simulink model "Clutchless_P2_Parallel"  (R2017b)
settings: Solver=FixedStepAuto  StartTime=0.0  StopTime=length(Speed)  FixedStep=0.01  MaxStep=0.01  RelTol=1e-3  EnableMultiTasking=on
PostLoadFcn:
  | , if any(exist('dsrtsu_mdlpostloadfcn', 'file') == [2, 3, 6]), try dsrtsu_mdlpostloadfcn('Execute', bdroot); catch fprintf('Error in PostLoadFcn (dsrtsu_mdlpostloadfcn) for model "%s":\n %s\n', bdroot, lasterr); end, end,
undefined symbols (not defined in the file): Actuators, APP1_OOR, APP2_OOR, APP_Mismatch, Brk_Flt, cal, Chassis, ClutchEngag, Clutchless_HSC, eng, Engine, EngineTorqueReal, EngOverTemp, ENGTRQ_MSMCH_Degraded_CP, ENGTRQ_MSMCH_ErrCritical_CP, ENGTRQ_MSMCH_LimpHome_CP, EngTrqMismatch, ess, ESSOverTemp, g, gb, Grade, KeyPos_Flt, lib_Actuators, lib_Chassis, lib_Clutchless_HSC, lib_EMachine_2017a, lib_Sensors_2017a, LossCAN, Machine, MCUOverTemp, mot, MotDirMismatch, motor_Trq, MotOverTemp, MotTrqMismatch, mph2ms, PRNDL_Flt, RegenFault, rho, Sensors, t_amb, time, tloop, veh, Vehicle
libraries: simulink x96, EC2_libraries x6, autolibmappedmotor x3, powerlib_meascontrol x2, CalculationGallon x1, lib_DCDC x1, lib_Differential x1, lib_HVESS x1, lib_Engine x1, lib_OBC x1, Scope_new x1, lib_Transmission x1
(part 4 of 10)

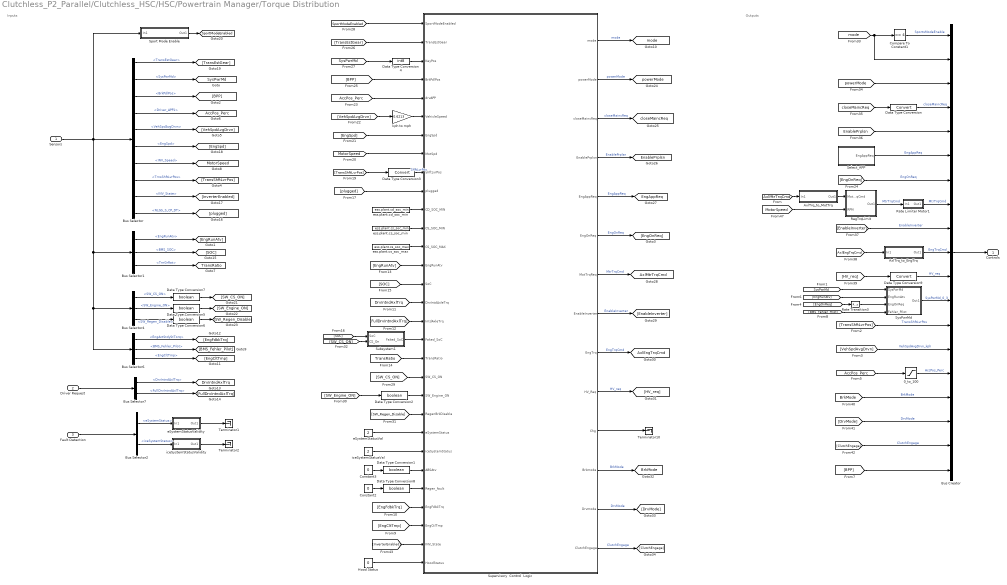
== system Clutchless_P2_Parallel/Clutchless_HSC/HSC/Powertrain Manager/Torque Distribution ==
  note: Inputs
  note: Outputs
  Sensors : Inport
  Driver Request : Inport  Port=2
  Fault Detection : Inport  Port=3
  0_to_100 : Saturate  UpperLimit=100  LowerLimit=0
  AxlTrq_to_EngTrq : Subsystem
  AxlTrq_to_MotTrq : Subsystem
  Bus Creator : BusCreator  Inputs=19
  Bus Selector : BusSelector  OutputSignals=from_CAN.fromVEH_CAN.from_TCM.TransEstGear,from_CAN.fromVEH_CAN.from_BCM.SysPwrMd,from_CAN.fromVEH_CAN.from_BCM.BrkPdlPos,from_Analog.Driver_APP1,from_CAN.fromEBCAN.from_ECM.VehSpdAvgDrvn,from_CAN.fromEBCAN.from_ECM.EngSpd,from_CAN.fromHV_CAN.from_MCU.INV_VCU_01.INV_Speed,from_CAN.fromVEH_CAN.from_TCM.TrnsShftLvrPos,from_CAN.fromHV_CAN.from_MCU.INV_VCU_01.INV_State,from_CAN.fromHV_CAN.from_OBC.NLG5_ST.NLG5_S_CP_DT
  Bus Selector1 : BusSelector  OutputSignals=from_CAN.fromEBCAN.from_ECM.EngRunAtv,from_CAN.fromHV_CAN.from_BMSHybrid.BMS_SOC,from_CAN.fromVEH_CAN.from_TCM.TrnGrRat
  Bus Selector2 : BusSelector  OutputSignals=eSystemDiagOut.eSystemStatus,iceSystemDiagOut.iceSystemStatus
  Bus Selector4 : BusSelector  OutputSignals=from_Digital.SW_CS_ON,from_Digital.SW_Engine_ON,from_Digital.SW_Regen_Disable
  Bus Selector6 : BusSelector  OutputSignals=from_CAN.fromEBCAN.from_ECM.EngActStdyStTorq,from_CAN.fromHV_CAN.from_BMSHybrid.BMS_HYB_02.BMS_Fehler_Pilot,from_CAN.fromEBCAN.from_ECM.EngCltTmp
  Bus Selector7 : BusSelector  OutputSignals=DrvIntndAxlTrq,FullDrvIntndAxlTrq
  Compare To Constant1 : simulink/Logic and Bit Operations/Compare To Constant  relop===  const=4  OutDataTypeStr=boolean
  Constant2 : Constant  Value=0
  Constant3 : Constant  Value=0
  Data Type Conversion : DataTypeConversion
  Data Type Conversion{1..2,5..8} (6 alike) : DataTypeConversion  OutDataTypeStr=boolean
  Data Type Conversion3 : DataTypeConversion
  Data Type Conversion4 : DataTypeConversion  OutDataTypeStr=int8
  Data Type Conversion9 : DataTypeConversion
  Hood Status : Constant  Value=0
  Rate Limiter Motor1 : Subsystem
  Rate Transition3 : RateTransition
  RegTrqLimit : Subsystem
  Select_APP : Subsystem
  Sport Mode Enable : Subsystem
  Subsystem1 : Subsystem
  Supervisory  Control  Logic : Stateflow chart  TreatAsAtomicUnit=on
  SysPwrMd : Subsystem
  Terminator1 : Terminator
  Terminator10 : Terminator
  Terminator2 : Terminator
  eSystemStatusVal : Constant  Value=2
  eSystemStatusValidity : Subsystem
  ess.plant.cd_soc_min : Constant  Value=ess.plant.cd_soc_min
  ess.plant.cs_soc_max : Constant  Value=ess.plant.cs_soc_max
  ess.plant.cs_soc_min : Constant  Value=ess.plant.cs_soc_min
  iceSystemStatusVal : Constant  Value=2
  iceSystemStatusValidity : Subsystem
  kph to mph : Gain  Gain=0.6213
  Controls : Outport
  tag scope: AccPos_Perc=global, AxlEngTrqCmd=global, AxlMtrTrqCmd=global, BrkMode=global, DrvIntndAxlTrq=global, EnablePrplsn=global, EngAppReq=global, MotorSpeed=global, SportModeEnabled=global, SysPwrMd=global, TransRatio=global, closeMaincReq=global, mode=global, powerMode=global
  wires:
  AxlTrq_to_MotTrq/1(Out1) -> RegTrqLimit/1(MotTrqCmd)
  [AxlMtrTrqCmd] -> AxlTrq_to_MotTrq/1(In1)
  [MotorSpeed] -> RegTrqLimit/2(RPM)
  Hood Status/1 -> Supervisory  Control  Logic/30(HoodStatus)
  [plugged] -> Supervisory  Control  Logic/10(plugged)
  AxlTrq_to_EngTrq/1(Out1) -> Bus Creator/10  "EngTrqCmd"
  [closeMaincReq] -> Data Type Conversion/1
  Compare To Constant1/1 -> Bus Creator/1  "SportsModeEnable"
  [EngRunAtv] -> SysPwrMd/2(EngRunAtv)
  [ClutchEngage] -> Bus Creator/18  "ClutchEngage"
  [BPP] -> Bus Creator/19
  [AxlEngTrqCmd] -> AxlTrq_to_EngTrq/1(In1)
  [mode] -> Compare To Constant1/1, Bus Creator/2
  [TransShftLvrPos] -> Bus Creator/13  "TransShftLvrPos"
  [DrvMode] -> Bus Creator/17  "DrvMode"
  [SysPwrMd] -> SysPwrMd/1(SysPwrMd)
  SysPwrMd/1(Out1) -> Bus Creator/12  "SysPwrMd_0_3"
  [VehSpdAvgDrvn] -> Bus Creator/14  "VehSpdAvgDrvn_kph"
  Data Type Conversion9/1 -> Bus Creator/11  "HV_req"
  [BMS_Fehler_Pilot] -> SysPwrMd/4(Fehler_Pilot)
  [EnablePrplsn] -> Bus Creator/5
  [AccPos_Perc] -> 0_to_100/1
  [EnableInverter] -> Bus Creator/9  "EnableInverter"
  [EngOnReq] -> Bus Creator/7  "EngOnReq"
  [HV_req] -> Data Type Conversion9/1
  Select_APP/1(EngAppReq) -> Bus Creator/6  "EngAppReq"
  [BrkMode] -> Bus Creator/16  "BrkMode"
  0_to_100/1 -> Bus Creator/15  "AccPos_Perc"
  [powerMode] -> Bus Creator/3
  Data Type Conversion/1 -> Bus Creator/4  "closeMaincReq"
  [EngOnReq] -> Rate Transition3/1
  Rate Transition3/1 -> SysPwrMd/3(EngOnReq)
  Bus Creator/1 -> Controls/1
  Sensors/1 -> Bus Selector/1, Bus Selector1/1, Bus Selector4/1, Bus Selector6/1, Sport Mode Enable/1(In1)
  Bus Selector/1 -> [TransEstGear]  "<TransEstGear>"
  Bus Selector/2 -> [SysPwrMd]  "<SysPwrMd>"
  Bus Selector/3 -> [BPP]  "<BrkPdlPos>"
  Bus Selector/4 -> [AccPos_Perc]  "<Driver_APP1>"
  Bus Selector/5 -> [VehSpdAvgDrvn]  "<VehSpdAvgDrvn>"
  Bus Selector/6 -> [EngSpd]  "<EngSpd>"
  Bus Selector/7 -> [MotorSpeed]  "<INV_Speed>"
  Bus Selector/9 -> [InverterEnabled]  "<INV_State>"
  Bus Selector1/1 -> [EngRunAtv]  "<EngRunAtv>"
  Bus Selector/8 -> [TransShftLvrPos]  "<TrnsShftLvrPos>"
  Bus Selector1/3 -> [TransRatio]  "<TrnGrRat>"
  Fault Detection/1 -> Bus Selector2/1
  Bus Selector2/1 -> eSystemStatusValidity/1(In1)  "<eSystemStatus>"
  Bus Selector2/2 -> iceSystemStatusValidity/1(In1)  "<iceSystemStatus>"
  Bus Selector4/3 -> Data Type Conversion6/1  "<SW_Regen_Disable>"
  Bus Selector4/1 -> Data Type Conversion7/1  "<SW_CS_ON>"
  Bus Selector4/2 -> Data Type Conversion5/1  "<SW_Engine_ON>"
  eSystemStatusValidity/1(Out1) -> Terminator1/1
  iceSystemStatusValidity/1(Out1) -> Terminator2/1
  Bus Selector/10 -> [plugged]  "<NLG5_S_CP_DT>"
  Data Type Conversion5/1 -> [SW_Engine_ON]
  Data Type Conversion6/1 -> [SW_Regen_Disable]
  Bus Selector6/1 -> [EngFdbkTrq]  "<EngActStdyStTorq>"
  Bus Selector6/2 -> [BMS_Fehler_Pilot]  "<BMS_Fehler_Pilot>"
  Bus Selector6/3 -> [EngCltTmp]  "<EngCltTmp>"
  Bus Selector7/2 -> [FullDrvIntndAxlTrq]  "<FullDrvIntndAxlTrq>"
  Sport Mode Enable/1(Out1) -> [SportModeEnabled]
  Bus Selector1/2 -> [SOC]  "<BMS_SOC>"
  Data Type Conversion7/1 -> [SW_CS_ON]
  Driver Request/1 -> Bus Selector7/1
  Bus Selector7/1 -> [DrvIntndAxlTrq]  "<DrvIntndAxlTrq>"
  Supervisory  Control  Logic/14(ClutchEngage) -> [ClutchEngage]  "ClutchEngage"
  Supervisory  Control  Logic/13(Drvmode) -> [DrvMode]  "DrvMode"
  Supervisory  Control  Logic/10(HV_Req) -> [HV_req]  "HV_req"
  Supervisory  Control  Logic/9(EngTrq) -> [AxlEngTrqCmd]  "EngTrqCmd"
  Supervisory  Control  Logic/7(MotTrqReq) -> [AxlMtrTrqCmd]  "MtrTrqCmd"
  Supervisory  Control  Logic/6(EngOnReq) -> [EngOnReq]  "EngOnReq"
  [SW_CS_ON] -> Subsystem1/2(CS_On)
  [SW_Regen_Disable] -> Supervisory  Control  Logic/22(RegenBrkDisable)
  [SW_CS_ON] -> Supervisory  Control  Logic/20(SW_CS_ON)
  [SportModeEnabled] -> Supervisory  Control  Logic/1(SportModeEnabled)
  Data Type Conversion4/1 -> Supervisory  Control  Logic/3(KeyPos)
  [SysPwrMd] -> Data Type Conversion4/1
  [TransEstGear] -> Supervisory  Control  Logic/2(TransEstGear)
  [BPP] -> Supervisory  Control  Logic/4(BrkPdlPos)
  [AccPos_Perc] -> Supervisory  Control  Logic/5(drvAPP)
  [VehSpdAvgDrvn] -> kph to mph/1
  [EngSpd] -> Supervisory  Control  Logic/7(EngSpd)
  [TransShftLvrPos] -> Data Type Conversion3/1
  [SOC] -> Subsystem1/1(SoC)
  [SOC] -> Supervisory  Control  Logic/15(SoC)
  [TransRatio] -> Supervisory  Control  Logic/19(TransRatio)
  [EngRunAtv] -> Supervisory  Control  Logic/14(EngRunAtv)
  [EngFdbkTrq] -> Supervisory  Control  Logic/27(EngFdbkTrq)
  [EngCltTmp] -> Supervisory  Control  Logic/28(EngCtlTmp)
  [MotorSpeed] -> Supervisory  Control  Logic/8(MotSpd)
  Supervisory  Control  Logic/5(EngAppReq) -> [EngAppReq]  "EngAppReq"
  eSystemStatusVal/1 -> Supervisory  Control  Logic/23(eSystemStatus)
  iceSystemStatusVal/1 -> Supervisory  Control  Logic/24(iceSystemStatus)
  Data Type Conversion8/1 -> Supervisory  Control  Logic/26(Regen_fault)
  Supervisory  Control  Logic/12(Brkmode) -> [BrkMode]  "BrkMode"
  Subsystem1/1(Faked_SoC) -> Supervisory  Control  Logic/18(Faked_SoC)
  Data Type Conversion1/1 -> Supervisory  Control  Logic/25(ABSAtv)
  Constant3/1 -> Data Type Conversion1/1
  [FullDrvIntndAxlTrq] -> Supervisory  Control  Logic/17(IntdAxleTrq)
  [DrvIntndAxlTrq] -> Supervisory  Control  Logic/16(DrvIntdAxleTrq)
  Supervisory  Control  Logic/11(Chg) -> Terminator10/1
  Constant2/1 -> Data Type Conversion8/1
  kph to mph/1 -> Supervisory  Control  Logic/6(VehicleSpeed)
  Data Type Conversion3/1 -> Supervisory  Control  Logic/9(ShftLvrPos)  "ShftLvrPos"
  Supervisory  Control  Logic/1(mode) -> [mode]  "mode"
  Supervisory  Control  Logic/2(powerMode) -> [powerMode]  "powerMode"
  Supervisory  Control  Logic/3(closeMaincReq) -> [closeMaincReq]  "closeMaincReq"
  Supervisory  Control  Logic/4(EnablePrplsn) -> [EnablePrplsn]  "EnablePrplsn"
  Supervisory  Control  Logic/8(EnableInverter) -> [EnableInverter]  "EnableInverter"
  ess.plant.cs_soc_max/1 -> Supervisory  Control  Logic/13(CS_SOC_MAX)
  ess.plant.cs_soc_min/1 -> Supervisory  Control  Logic/12(CS_SOC_MIN)
  ess.plant.cd_soc_min/1 -> Supervisory  Control  Logic/11(CD_SOC_MIN)
  [SW_Engine_ON] -> Data Type Conversion2/1
  Data Type Conversion2/1 -> Supervisory  Control  Logic/21(SW_Engine_ON)
  [InverterEnabled] -> Supervisory  Control  Logic/29(INV_State)
  RegTrqLimit/1(Out1) -> Rate Limiter Motor1/1(In1)  "MtrTrqCmd"
  Rate Limiter Motor1/1(Out1) -> Bus Creator/8  "MtrTrqCmd"

== system Clutchless_P2_Parallel/Sensors/CAN/EBCAN/BMS_Antrieb ==
  In1 : Inport
  Bus Creator : BusCreator  Inputs=2
  Bus Selector : BusSelector  OutputSignals=NMH_BMS,ISO_Hybrid_01_Resp
  ISO_Hybrid_01_Resp : Subsystem
  NMH_BMS : Subsystem
  Out1 : Outport
  wires:
  Bus Selector/2 -> ISO_Hybrid_01_Resp/1(In1)  "<ISO_Hybrid_01_Resp>"
  Bus Creator/1 -> Out1/1
  ISO_Hybrid_01_Resp/1(Out1) -> Bus Creator/2
  NMH_BMS/1(Out1) -> Bus Creator/1
  Bus Selector/1 -> NMH_BMS/1(In1)  "<NMH_BMS>"
  In1/1 -> Bus Selector/1

== system Clutchless_P2_Parallel/Sensors/CAN/EBCAN/CCM ==
  In1 : Inport
  Bus Creator : BusCreator  Inputs=2
  Bus Selector : BusSelector  OutputSignals=NMH_BMS,ISO_Hybrid_01_Resp
  ISO_Hybrid_01_Resp : Subsystem
  NMH_BMS : Subsystem
  Out1 : Outport
  wires:
  In1/1 -> Bus Selector/1
  Bus Selector/1 -> NMH_BMS/1(In1)  "<NMH_BMS>"
  NMH_BMS/1(Out1) -> Bus Creator/1
  ISO_Hybrid_01_Resp/1(Out1) -> Bus Creator/2
  Bus Creator/1 -> Out1/1
  Bus Selector/2 -> ISO_Hybrid_01_Resp/1(In1)  "<ISO_Hybrid_01_Resp>"

== system Clutchless_P2_Parallel/Sensors/CAN/EBCAN/ECM ==
  In1 : Inport
  Bus Creator : BusCreator  Inputs=7
  Bus Selector : BusSelector  OutputSignals=Sensors_to_ECM.EngActStdyStTorq_Nm,Sensors_to_ECM.EngSpd_RPM,ECM_to_Actuators.VehSpdAvgDrvn,ECM_to_Actuators.EngRunAtv,ECM_to_Actuators.Eng_Temp,ECM_to_Actuators.ECM_RollingAliveCnt
  Data Type Conversion{1..6} (6 alike) : DataTypeConversion
  ETEI_Engine_Torque_Status : Subsystem
  Ground : Ground
  PPEI_Engine_General_Status_4 : Subsystem
  PPEI_Engine_General_Status_6 : Subsystem
  PPEI_Vehicle_Speed_and_Distance : Subsystem
  PTEI_Engine_Torque_Status : Subsystem
  Out1 : Outport
  wires:
  Data Type Conversion1/1 -> Bus Creator/4  "EngRunAtv"
  Data Type Conversion3/1 -> Bus Creator/2  "EngSpd"
  PPEI_Engine_General_Status_6/1(Out1) -> Bus Creator/7
  Data Type Conversion6/1 -> PPEI_Engine_General_Status_6/1(In1)
  PPEI_Engine_General_Status_4/1(Out1) -> Bus Creator/6
  Data Type Conversion5/1 -> PPEI_Engine_General_Status_4/1(In1)
  PTEI_Engine_Torque_Status/1(Out1) -> Bus Creator/5
  Ground/1 -> PTEI_Engine_Torque_Status/1(In1)
  Bus Selector/4 -> Data Type Conversion1/1  "<EngRunAtv>"
  Bus Creator/1 -> Out1/1
  PPEI_Vehicle_Speed_and_Distance/1(Out1) -> Bus Creator/3
  ETEI_Engine_Torque_Status/1(Out1) -> Bus Creator/1
  Data Type Conversion4/1 -> PPEI_Vehicle_Speed_and_Distance/1(In1)
  Bus Selector/2 -> Data Type Conversion3/1  "<EngSpd_RPM>"
  Data Type Conversion2/1 -> ETEI_Engine_Torque_Status/1(In1)
  In1/1 -> Bus Selector/1
  Bus Selector/1 -> Data Type Conversion2/1  "<EngActStdyStTorq_Nm>"
  Bus Selector/3 -> Data Type Conversion4/1  "<VehSpdAvgDrvn>"
  Bus Selector/5 -> Data Type Conversion5/1  "<Eng_Temp>"
  Bus Selector/6 -> Data Type Conversion6/1  "<ECM_RollingAliveCnt>"

== system Clutchless_P2_Parallel/Sensors/CAN/HV_CAN/BMS_Hybrid ==
  In1 : Inport
  BMS_HYB_02 : Subsystem
  BMS_HYB_03 : Subsystem
  BMS_HYB_04 : Subsystem
  Bus Creator : BusCreator  Inputs=6
  Bus Selector : BusSelector  OutputSignals=BMS_HYB_02,BMS_HYB_04,BMS_HYB_03,BMS_HYB_02.BMS_Fehler_Isolation,BMS_HYB_06.BMS_Temperatur,BMS_HYB_02.BMS_Fehler_HS_verschweisst
  Data Type Conversion : DataTypeConversion
  Data Type Conversion1 : DataTypeConversion
  Data Type Conversion2 : DataTypeConversion
  Out1 : Outport
  wires:
  Data Type Conversion2/1 -> Bus Creator/6  "BMS_Fehler_HS_verschweisst"
  Bus Selector/5 -> Data Type Conversion/1  "<BMS_Temperatur>"
  Bus Selector/4 -> Data Type Conversion1/1  "<BMS_Fehler_Isolation>"
  BMS_HYB_03/1(Out1) -> Bus Creator/3
  Bus Selector/3 -> BMS_HYB_03/1(In1)  "<BMS_HYB_03>"
  BMS_HYB_04/1(Out1) -> Bus Creator/2
  BMS_HYB_02/1(Out1) -> Bus Creator/1
  Bus Creator/1 -> Out1/1
  Bus Selector/2 -> BMS_HYB_04/1(In1)  "<BMS_HYB_04>"
  Bus Selector/1 -> BMS_HYB_02/1(In1)  "<BMS_HYB_02>"
  In1/1 -> Bus Selector/1
  Data Type Conversion/1 -> Bus Creator/5  "BMS_Temperatur"
  Data Type Conversion1/1 -> Bus Creator/4  "BMS_Fehler_Isolation"
  Bus Selector/6 -> Data Type Conversion2/1  "<BMS_Fehler_HS_verschweisst>"

== system Clutchless_P2_Parallel/Sensors/CAN/HV_CAN/MCU ==
  In1 : Inport
  Bus Creator : BusCreator  Inputs=6
  Bus Creator1 : BusCreator  Inputs=2
  Bus Creator2 : BusCreator  Inputs=2
  Bus Selector : BusSelector  OutputSignals=Sensors_to_MCU.mot_spd_out,Sensors_to_MCU.mot_crr_out,MCU_to _Actuator.InverterEnabled,MCU_to _Actuator.MotTrqFdbck,MCU_to _Actuator.D3_Power_On_Timer,Sensors_to_MCU.mot_volt_in
  Bus Selector1 : BusSelector  OutputSignals=Sensors_to_MCU.mcu_temp,Sensors_to_MCU.mot_temp
  Data Type Conversion{1..5,7..9} (8 alike) : DataTypeConversion
  In2 : InportShadow
  Out1 : Outport
  wires:
  In1/1 -> Bus Selector/1
  Bus Selector/6 -> Data Type Conversion9/1  "<mot_volt_in>"
  Bus Selector/4 -> Data Type Conversion7/1  "<MotTrqFdbck>"
  Bus Selector/5 -> Data Type Conversion8/1  "<D3_Power_On_Timer>"
  Bus Creator/1 -> Bus Creator1/1  "INV_VCU_01"
  Data Type Conversion3/1 -> Bus Creator/3  "INV_State"
  Data Type Conversion2/1 -> Bus Creator/2  "INV_CurrentHV"
  Data Type Conversion1/1 -> Bus Creator/1  "INV_Speed"
  Bus Selector/3 -> Data Type Conversion3/1  "<InverterEnabled>"
  Bus Selector/2 -> Data Type Conversion2/1  "<mot_crr_out>"
  Bus Selector/1 -> Data Type Conversion1/1  "<mot_spd_out>"
  Data Type Conversion7/1 -> Bus Creator/4  "INV_OutputTorque"
  Data Type Conversion8/1 -> Bus Creator/5  "MessageCounter_200"
  Data Type Conversion9/1 -> Bus Creator/6  "INV_VoltageHV"
  Data Type Conversion4/1 -> Bus Creator2/1  "INV_InverterTemperature"
  Bus Selector1/2 -> Data Type Conversion5/1  "<mot_temp>"
  Data Type Conversion5/1 -> Bus Creator2/2  "INV_ElectricMachineTemperature"
  Bus Selector1/1 -> Data Type Conversion4/1  "<mcu_temp>"
  In2/1 -> Bus Selector1/1
  Bus Creator2/1 -> Bus Creator1/2  "INV_VCU_04"
  Bus Creator1/1 -> Out1/1

== system Clutchless_P2_Parallel/Sensors/CAN/HV_CAN/OBC ==
  In1 : Inport
  Bus Creator : BusCreator  Inputs=5
  Bus Selector : BusSelector  OutputSignals=NLG5_ACT_I,NLG5_ACT_II,NLG5_ERR,NLG5_ST,NLG5_TEMP
  NLG5_ACT_I : Subsystem
  NLG5_ACT_II : Subsystem
  NLG5_ERR : Subsystem
  NLG5_ST : Subsystem
  NLG5_TEMP : Subsystem
  Out1 : Outport
  wires:
  In1/1 -> Bus Selector/1
  Bus Selector/1 -> NLG5_ACT_I/1(In1)  "<NLG5_ACT_I>"
  NLG5_ACT_I/1(Out1) -> Bus Creator/1
  Bus Selector/2 -> NLG5_ACT_II/1(In1)  "<NLG5_ACT_II>"
  NLG5_ACT_II/1(Out1) -> Bus Creator/2
  NLG5_ERR/1(Out1) -> Bus Creator/3
  Bus Selector/3 -> NLG5_ERR/1(In1)  "<NLG5_ERR>"
  Bus Selector/4 -> NLG5_ST/1(In1)  "<NLG5_ST>"
  NLG5_ST/1(Out1) -> Bus Creator/4
  Bus Selector/5 -> NLG5_TEMP/1(In1)  "<NLG5_TEMP>"
  NLG5_TEMP/1(Out1) -> Bus Creator/5
  Bus Creator/1 -> Out1/1

== system Clutchless_P2_Parallel/Sensors/CAN/VEH_CAN/BCM ==
  In1 : Inport
  Bus Creator : BusCreator  Inputs=2
  Bus Selector : BusSelector  OutputSignals=SysPwrMd,BrkPdlPos
  Data Type Conversion : DataTypeConversion
  Data Type Conversion1 : DataTypeConversion
  PPEI_Brake_Apply_Status : Subsystem
  PPEI_Platfrom_General_Status : Subsystem
  Out1 : Outport
  wires:
  Data Type Conversion1/1 -> PPEI_Brake_Apply_Status/1(In1)
  Data Type Conversion/1 -> PPEI_Platfrom_General_Status/1(In1)
  Bus Creator/1 -> Out1/1
  PPEI_Brake_Apply_Status/1(Out1) -> Bus Creator/2
  PPEI_Platfrom_General_Status/1(Out1) -> Bus Creator/1
  Bus Selector/2 -> Data Type Conversion1/1  "<BrkPdlPos>"
  Bus Selector/1 -> Data Type Conversion/1  "<SysPwrMd>"
  In1/1 -> Bus Selector/1

== system Clutchless_P2_Parallel/Sensors/CAN/VEH_CAN/EBCM ==
  In1 : Inport
  Bus Selector : BusSelector  OutputSignals=PPEI_Chassis_General_Status_1.BrkPdlDrvAppPrsDetcd
  Constant : Constant  OutDataTypeStr=boolean
  PPEI_Chassis_General_Status_1 : Subsystem
  Terminator : Terminator
  Out1 : Outport
  wires:
  Constant/1 -> PPEI_Chassis_General_Status_1/1(In1)
  In1/1 -> Bus Selector/1
  PPEI_Chassis_General_Status_1/1(Out1) -> Out1/1
  Bus Selector/1 -> Terminator/1  "<BrkPdlDrvAppPrsDetcd>"

== system Clutchless_P2_Parallel/Sensors/CAN/VEH_CAN/ICCM ==
  In1 : Inport
  Out1 : Outport
  wires:
  In1/1 -> Out1/1

== system Clutchless_P2_Parallel/Sensors/CAN/VEH_CAN/TCM ==
  In1 : Inport
  Bus Creator : BusCreator  Inputs=4
  Bus Selector : BusSelector  OutputSignals=TCM_to _Actuator.TransEstGear,TCM_to _Actuator.LockupCmd,TCM_to _Actuator.TrnsShftLvrPos,Sensors_to_TCM.gb_trq_ratio
  Data Type Conversion{,1..3} (4 alike) : DataTypeConversion
  Out1 : Outport
  wires:
  Data Type Conversion/1 -> Bus Creator/1  "TransEstGear"
  Bus Creator/1 -> Out1/1
  In1/1 -> Bus Selector/1
  Data Type Conversion1/1 -> Bus Creator/2  "TrnsTrqCnvCltCmndMd"
  Data Type Conversion2/1 -> Bus Creator/3  "TrnsShftLvrPos"
  Data Type Conversion3/1 -> Bus Creator/4  "TrnGrRat"
  Bus Selector/1 -> Data Type Conversion/1  "<TransEstGear>"
  Bus Selector/2 -> Data Type Conversion1/1  "<LockupCmd>"
  Bus Selector/3 -> Data Type Conversion2/1  "<TrnsShftLvrPos>"
  Bus Selector/4 -> Data Type Conversion3/1  "<gb_trq_ratio>"

== system Clutchless_P2_Parallel/Camaro Plant Model/E-Machine/IMG Plant/Electric Machine/Calculate Mot Efficiency, MotPwrMech, and, MotPwrElec1 ==
  note: Pelec_req = Pmech_req*Eff^k,
      | k = -1 if Trq >= 0,
      | k = 1 if Trq < 0
  MotSpd : Inport
  MotTrqAct : Inport  Port=2
  -1 : Gain  Gain=8
  "-1 when + 1 when - " : Gain  Gain=-1
  -2 : Gain  Gain=tloop
  2-D Lookup Table : Lookup_n-D  BreakpointsForDimension1=mot.plant.init.eff_trq.idx2_trq  BreakpointsForDimension2=mot.plant.init.eff_trq.idx1_spd  Table=mot.plant.init.eff_trq.map  InternalRulePriority=Speed  RndMeth=Simplest  InputSameDT=on
  Abs{,1..3} (4 alike) : Abs
  Add : Sum  Inputs=-+
  Add1 : Sum  Inputs=+-
  Constant : Constant  Value=1-0.8
  Gain2 : Gain  Gain=1/100
  MCU_WEGPmp : Constant  Value=0
  Math Function1 : Math  Operator=pow  SaturateOnIntegerOverflow=on
  Memory : Memory
  Product : Product
  Product1 : Product
  Product2 : Product
  Sign : Signum
  rad/s to rpm : Gain  Gain=30/pi
  Losses : Outport
  MCU_Heat : Outport  Port=2
  MotPwrElec : Outport  Port=3
  wires:
  -2/1 -> MCU_Heat/1
  -1/1 -> Add1/2
  Add1/1 -> -2/1
  MCU_WEGPmp/1 -> -1/1
  Abs3/1 -> Add1/1
  Product2/1 -> Abs3/1
  Constant/1 -> Product2/2
  Memory/1 -> Sign/1
  Math Function1/1 -> Product1/2
  Add/1 -> Abs2/1
  Abs2/1 -> Losses/1
  "-1 when + 1 when - "/1 -> Math Function1/2
  MotSpd/1 -> rad/s to rpm/1, Product/2
  MotTrqAct/1 -> Abs/1, Product/1, Memory/1
  Product/1 -> Product1/1, Add/1  "MotPwrMech"
  Product1/1 -> Add/2, Product2/1, MotPwrElec/1  "MotPwrElec"
  2-D Lookup Table/1 -> Gain2/1
  Gain2/1 -> Math Function1/1
  Abs/1 -> 2-D Lookup Table/1
  Sign/1 -> "-1 when + 1 when - "/1
  Abs1/1 -> 2-D Lookup Table/2
  rad/s to rpm/1 -> Abs1/1

== system Clutchless_P2_Parallel/Camaro Plant Model/E-Machine/IMG Plant/Electric Machine/MotTrqExcessTrigger1 ==
  In1 : Inport
  Bias : Bias  Bias=55
  Bias1 : Bias  Bias=25
  Constant : Constant  Value=0
  Multiport Switch : MultiPortSwitch  DataPortOrder=Zero-based contiguous
  Terminator : Terminator
  Out1 : Outport
  tag scope: MotTrqExcessTrig=global
  wires:
  Constant/1 -> Multiport Switch/1, [MotTrqExcessTrig]
  Bias1/1 -> Multiport Switch/3
  In1/1 -> Bias1/1, Bias/1, Multiport Switch/2
  Bias/1 -> Multiport Switch/4
  Multiport Switch/1 -> Out1/1
  [MotTrqExcessTrig] -> Terminator/1

== system Clutchless_P2_Parallel/Camaro Plant Model/E-Machine/IMG Plant/Electric Machine/Thermal1 ==
  Losses : Inport
  MCU_heat : Inport  Port=2
  MotInv_loop : Subsystem
  Motor Thermal : Subsystem  Commented=on
  MCU_temp_C : Outport
  motor_temp : Outport  Port=2
  wires:
  MotInv_loop/2(Out2) -> motor_temp/1
  MotInv_loop/1(Out1) -> MCU_temp_C/1
  Losses/1 -> MotInv_loop/1(In1)  "[W]"
  MCU_heat/1 -> MotInv_loop/2(In2)

== system Clutchless_P2_Parallel/Camaro Plant Model/E-Machine/IMG Plant/Electric Machine/Torque Calculation1 ==
  MotSpd : Inport
  MotTrqCmd : Inport  Port=2
  Abs : Abs
  Abs1 : Abs
  Memory : Memory
  MinMax : MinMax  Inputs=2
  Product : Product
  Sign : Signum
  "max torque " : Subsystem
  mot_trq_out : Outport
  wires:
  Product/1 -> Memory/1
  MotTrqCmd/1 -> Abs/1, Sign/1, "max torque "/1(cmd)
  Memory/1 -> mot_trq_out/1
  Abs1/1 -> MinMax/2
  Abs/1 -> MinMax/1
  MinMax/1 -> Product/2
  Sign/1 -> Product/1
  MotSpd/1 -> "max torque "/2(speed)
  "max torque "/1(max torque) -> Abs1/1

== system Clutchless_P2_Parallel/Camaro Plant Model/E-Machine/IMG Plant/Electric Machine/non-zero division1 ==
  note: and finally, the expression is: (u[1] \ u[2]) * 1 = u[1] \ u[2]
  note: (u[2]!=0) is true then returns 1
  note: if u[2] != 0, then output == u[1]\u[2]:
  note: (u[2]==0) is false then returns 0, thus (u[2]+(u[2]==0)) is equal to u[2]+0=u[2]
  note: and finally, the expression is: (u[1] \ 1) * 0 = 0
  note: (u[2]!=0) is false then returns 0
  note: if u[2] == 0, then output == 0:
  note: (u[2]==0) is true then returns 1, thus (u[2]+(u[2]==0)) is equal to 0+1=1
  note: original idea from Phil Sharer - ANL
      | original formula: u[1]\(u[2]+eps)*(u[2]!=0)
      | changes done by Gerald ZINI (dgey) - ANL (05\02\2001)
  In1 : Inport
  In2 : Inport  Port=2
  Fcn : Fcn  Expr=u[1]/(u[2]+(u[2]==0))*(u[2]!=0)
  Mux : Mux  Inputs=2
  Out1 : Outport
  wires:
  In2/1 -> Mux/2
  Fcn/1 -> Out1/1
  In1/1 -> Mux/1
  Mux/1 -> Fcn/1

== system Clutchless_P2_Parallel/Camaro Plant Model/E-Machine/IMG Plant2/Calculate Mot Efficiency, MotPwrMech, and, MotPwrElec/Lower Limit ==
  In1 : Inport
  Constant3 : Constant  Value=Lolimit
  MinMax : MinMax  Function=max  Inputs=2
  Out1 : Outport
  wires:
  MinMax/1 -> Out1/1
  Constant3/1 -> MinMax/2
  In1/1 -> MinMax/1

== system Clutchless_P2_Parallel/Camaro Plant Model/E-Machine/IMG Plant2/Calculate Mot Efficiency, MotPwrMech, and, MotPwrElec/MCUOverTemp Fault ==
  In1 : Inport
  Gain : Gain  Gain=3
  Switch : Switch  Threshold=1
  Out1 : Outport
  wires:
  Switch/1 -> Out1/1
  Gain/1 -> Switch/1
  [MCUOverTemp] -> Switch/2
  In1/1 -> Gain/1, Switch/3

== system Clutchless_P2_Parallel/Camaro Plant Model/E-Machine/IMG Plant2/Motor_Plant/Efficiency Calcs ==
  Speed_rpm : Inport
  Torq_cmd_Nm : Inport  Port=2
  Batt_volt : Inport  Port=3
  Abs1 : Abs
  Constant : Constant
  Constant1 : Constant  Value=0
  Current_consum : Product  Inputs=*/
  Efficiency Map : Lookup_n-D  BreakpointsForDimension1=mot.map.trqindex  BreakpointsForDimension2=mot.map.spdindex  Table=mot.map.eff  InternalRulePriority=Speed  RndMeth=Simplest  InputSameDT=on
  Electrical power motoring : Product  Inputs=*//
  Electrical power regen : Product  Inputs=***
  Gain : Gain  Gain=2*3.14/60
  Gain1 : Gain  Gain=-1
  MCU_eff : Constant  Value=0.97
  Mech_power : Product  Inputs=**
  MinMax : MinMax  Function=max  Inputs=2
  MinMax1 : MinMax  Function=max  Inputs=2
  Saturation : Saturate  UpperLimit=400  LowerLimit=-400
  Switch : Switch  Criteria=u2 > Threshold
  Switch1 : Switch  Criteria=u2 > Threshold  Threshold=100
  min_eff : Constant  Value=0.1
  Mot_current : Outport
  Mech_power_W : Outport  Port=2
  Elec_power_W : Outport  Port=3
  wires:
  Constant1/1 -> Switch1/3
  Switch/1 -> Switch1/1  "Elec_power_W"
  Gain1/1 -> Saturation/1  "Mot_current_A"
  Constant/1 -> MinMax1/2
  MinMax1/1 -> Current_consum/2
  Efficiency Map/1 -> MinMax/1
  Switch1/1 -> Current_consum/1, Elec_power_W/1  "Elec_power_W"
  min_eff/1 -> MinMax/2
  Electrical power motoring/1 -> Switch/1
  MCU_eff/1 -> Electrical power motoring/3, Electrical power regen/3
  Mech_power/1 -> Mech_power_W/1, Electrical power regen/1, Electrical power motoring/1  "Mech_power_W"
  Abs1/1 -> Efficiency Map/1
  Batt_volt/1 -> MinMax1/1, Switch1/2
  Gain/1 -> Mech_power/1
  Saturation/1 -> Mot_current/1  "Mot_current_A"
  Current_consum/1 -> Gain1/1
  MinMax/1 -> Electrical power regen/2, Electrical power motoring/2
  Electrical power regen/1 -> Switch/3
  Torq_cmd_Nm/1 -> Switch/2, Abs1/1, Mech_power/2
  Speed_rpm/1 -> Gain/1, Efficiency Map/2

== system Clutchless_P2_Parallel/Camaro Plant Model/E-Machine/IMG Plant2/Thermal/Motor Thermal ==
  In1 : Inport
  Add1 : Sum  Inputs=+-
  Add2 : Sum
  Divide : Product  Inputs=*/
  Lower Limit : Subsystem  mask{Lolimit=t_amb+20}
      mask prompts: Lolimit "Lower Limit"
  Memory1 : Memory
  Motor Mass : Constant  Value=mot.plant.init.motor_mass
  Product : Product  RndMeth=Zero
  "Pump " : Constant  Value=0
  Specific Heat Cap Aluminum : Constant  Value=mot.plant.init.specific_heat
  tloop : Gain  Gain=tloop
  Out1 : Outport
  wires:
  Add1/1 -> tloop/1
  In1/1 -> Add1/1
  "Pump "/1 -> Add1/2
  Motor Mass/1 -> Product/1  "kg"
  tloop/1 -> Divide/1  "J"
  Divide/1 -> Add2/1
  Lower Limit/1(Out1) -> Memory1/1, Out1/1
  Add2/1 -> Lower Limit/1(In1)
  Memory1/1 -> Add2/2
  Product/1 -> Divide/2
  Specific Heat Cap Aluminum/1 -> Product/2  "J/kg*K"

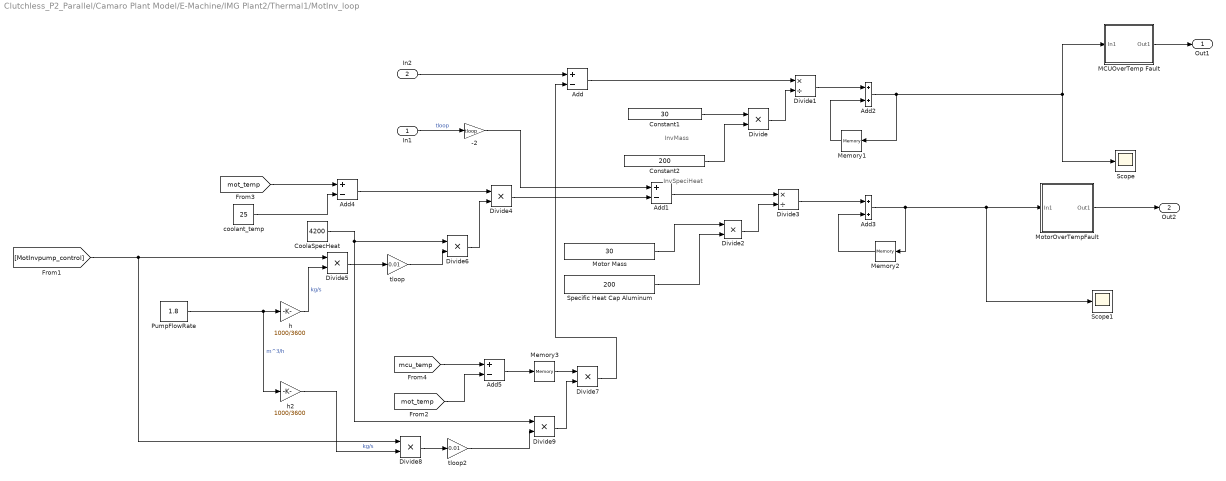
== system Clutchless_P2_Parallel/Camaro Plant Model/E-Machine/IMG Plant2/Thermal1/MotInv_loop ==
  note: InvMass
  note: InvSpeciHeat
  In1 : Inport
  In2 : Inport  Port=2
  -2 : Gain  Gain=tloop
  Add{,1,4..5} (4 alike) : Sum  Inputs=+-
  Add2 : Sum
  Add3 : Sum
  Constant1 : Constant  Value=30
  Constant2 : Constant  Value=200
  CoolaSpecHeat : Constant  Value=4200
  Divide{,2,4..9} (8 alike) : Product  Inputs=**
  Divide1 : Product  Inputs=*/
  Divide3 : Product  Inputs=*/
  MCUOverTemp Fault : Subsystem
  Memory1 : Memory  InitialCondition=25
  Memory2 : Memory  InitialCondition=25
  Memory3 : Memory
  Motor Mass : Constant  Value=30
  MotorOverTempFault : Subsystem
  PumpFlowRate : Constant  Value=1.8
  Scope : Scope
  Scope1 : Scope
  Specific Heat Cap Aluminum : Constant  Value=200
  coolant_temp : Constant  Value=25
  h : Gain  Gain=1000/3600
  h2 : Gain  Gain=1000/3600
  tloop : Gain  Gain=0.01
  tloop2 : Gain  Gain=0.01
  Out1 : Outport
  Out2 : Outport  Port=2
  wires:
  [MotInvpump_control] -> Divide5/1, Divide8/1
  -2/1 -> Add1/1
  In2/1 -> Add/1
  In1/1 -> -2/1  "tloop"
  [mot_temp] -> Add5/2
  [mcu_temp] -> Add5/1
  [mot_temp] -> Add4/1
  MotorOverTempFault/1(Out1) -> Out2/1
  MCUOverTemp Fault/1(Out1) -> Out1/1
  Memory3/1 -> Divide7/1
  Add5/1 -> Memory3/1
  Divide4/1 -> Add1/2
  tloop2/1 -> Divide9/2
  Divide8/1 -> tloop2/1
  Divide9/1 -> Divide7/2
  h2/1 -> Divide8/2  "kg/s"
  PumpFlowRate/1 -> h/1, h2/1  "m^3/h"
  CoolaSpecHeat/1 -> Divide9/1, Divide6/1
  tloop/1 -> Divide6/2
  h/1 -> Divide5/2  "kg/s"
  Divide7/1 -> Add/2
  Divide1/1 -> Add2/1
  Motor Mass/1 -> Divide2/1
  Constant2/1 -> Divide/2
  Divide2/1 -> Divide3/2
  Add2/1 -> Memory1/1, Scope/1, MCUOverTemp Fault/1(In1)
  Divide5/1 -> tloop/1
  Divide3/1 -> Add3/1
  Divide6/1 -> Divide4/2
  Add3/1 -> Memory2/1, MotorOverTempFault/1(In1), Scope1/1
  Add4/1 -> Divide4/1
  Memory2/1 -> Add3/2
  Add/1 -> Divide1/1
  Constant1/1 -> Divide/1
  Specific Heat Cap Aluminum/1 -> Divide2/2
  Divide/1 -> Divide1/2
  coolant_temp/1 -> Add4/2
  Memory1/1 -> Add2/2
  Add1/1 -> Divide3/1

== system Clutchless_P2_Parallel/Camaro Plant Model/E-Machine/IMG Plant2/Thermal1/Motor Thermal ==
  In1 : Inport
  Add1 : Sum  Inputs=+-
  Add2 : Sum
  Divide : Product  Inputs=*/
  Lower Limit : Subsystem  mask{Lolimit=t_amb+20}
      mask prompts: Lolimit "Lower Limit"
  Memory1 : Memory
  Motor Mass : Constant  Value=mot.plant.init.motor_mass
  Product : Product  RndMeth=Zero
  "Pump " : Constant  Value=0
  Specific Heat Cap Aluminum : Constant  Value=mot.plant.init.specific_heat
  tloop : Gain  Gain=tloop
  Out1 : Outport
  wires:
  Add1/1 -> tloop/1
  In1/1 -> Add1/1
  "Pump "/1 -> Add1/2
  Motor Mass/1 -> Product/1  "kg"
  tloop/1 -> Divide/1  "J"
  Divide/1 -> Add2/1
  Lower Limit/1(Out1) -> Memory1/1, Out1/1
  Add2/1 -> Lower Limit/1(In1)
  Memory1/1 -> Add2/2
  Product/1 -> Divide/2
  Specific Heat Cap Aluminum/1 -> Product/2  "J/kg*K"

== system Clutchless_P2_Parallel/Camaro Plant Model/E-Machine/IMG Plant2/Torque Calculation/electric machine filter ==
  trq : Inport
  Interval Test : simulink/Logic and Bit Operations/Interval Test  IntervalClosedRight=on  uplimit=0.5  IntervalClosedLeft=on  lowlimit=-0.5  OutDataTypeStr=boolean
  Switch : Switch  Threshold=0.5
  electric machine time response : TransferFcn  Denominator=[mot.plant.init.time_response 1]
  filtered : Outport
  wires:
  Switch/1 -> filtered/1
  trq/1 -> Switch/1, electric machine time response/1, Interval Test/1
  Interval Test/1 -> Switch/2
  electric machine time response/1 -> Switch/3

== system Clutchless_P2_Parallel/Camaro Plant Model/E-Machine/IMG Plant2/Torque Calculation/max torque  ==
  cmd : Inport
  speed : Inport  Port=2
  Memory : Memory
  Peak trq max - Motoring : Lookup  InputValues=mot.plant.init.regen.trq_max.idx1_spd  Table=mot.plant.init.motor.trq_max.map  LookUpMeth=Interpolation-Use End Values  SaturateOnIntegerOverflow=on
  Peak trq max - Regen : Lookup  InputValues=mot.plant.init.regen.trq_max.idx1_spd  Table=mot.plant.init.regen.trq_max.map  LookUpMeth=Interpolation-Use End Values  SaturateOnIntegerOverflow=on
  Switch1 : Switch  SaturateOnIntegerOverflow=on
  rad/s  to RPM : Gain  Gain=30/pi
  max torque : Outport
  wires:
  Peak trq max - Regen/1 -> Switch1/3
  rad/s  to RPM/1 -> Memory/1
  Memory/1 -> Peak trq max - Regen/1, Peak trq max - Motoring/1
  Switch1/1 -> max torque/1
  cmd/1 -> Switch1/2
  speed/1 -> rad/s  to RPM/1
  Peak trq max - Motoring/1 -> Switch1/1

== system Clutchless_P2_Parallel/Camaro Plant Model/E-Machine/Soft MCU/Subsystem/MCU_RollingAliveCnt ==
  Counter Free-Running : simulink/Sources/Counter Free-Running  NumBits=4  tsamp=-1
  Out1 : Outport
  wires:
  Counter Free-Running/1 -> Out1/1  "MCURollingAliveCnt [0 1 2 3]"

== system Clutchless_P2_Parallel/Camaro Plant Model/E-Machine/Soft MCU/Torque Calculation1/max torque  ==
  Req : Inport
  speed : Inport  Port=2
  torque : Inport  Port=3
  2-D Lookup Table : Lookup_n-D  Commented=on  BreakpointsForDimension1=mot.plant.init.eff_trq.idx2_trq  BreakpointsForDimension2=mot.plant.init.eff_trq.idx1_spd  Table=mot.plant.init.eff_trq.map  InternalRulePriority=Speed  RndMeth=Simplest  InputSameDT=on
  Abs : Abs  SaturateOnIntegerOverflow=on
  Abs1 : Abs  Commented=on
  Abs2 : Abs  Commented=on
  Constant : Constant  Commented=on  Value=84500
  Cont trq max - Motoring : Lookup  InputValues=mot.plant.init.motor.trq_cont.idx1_spd  Table=mot.plant.init.motor.trq_cont.map  LookUpMeth=Interpolation-Use End Values  SaturateOnIntegerOverflow=on
  Cont trq max - Regen : Lookup  InputValues=mot.plant.init.regen.trq_cont.idx1_spd  Table=mot.plant.init.regen.trq_cont.map  LookUpMeth=Interpolation-Use End Values  SaturateOnIntegerOverflow=on
  Divide : Product  Commented=on  Inputs=**/
  Divide by zero : Subsystem  Commented=on
  Gain2 : Gain  Commented=on  Gain=1/100
  Heat index : Subsystem
  Memory : Memory
  Peak trq max - Motoring : Lookup  Commented=on  InputValues=mot.plant.init.regen.trq_max.idx1_spd  Table=mot.plant.init.motor.trq_max.map  LookUpMeth=Interpolation-Use End Values  SaturateOnIntegerOverflow=on
  Peak trq max - Motoring1 : Lookup  InputValues=mot.plant.init.regen.trq_max.idx1_spd  Table=mot.plant.init.motor.trq_max.map  LookUpMeth=Interpolation-Use End Values  SaturateOnIntegerOverflow=on
  Peak trq max - Regen : Lookup  InputValues=mot.plant.init.regen.trq_max.idx1_spd  Table=mot.plant.init.regen.trq_max.map  LookUpMeth=Interpolation-Use End Values  SaturateOnIntegerOverflow=on
  Product2 : Product  SaturateOnIntegerOverflow=on  InputSameDT=on  OutDataTypeStr=Inherit: Same as first input
  Product3 : Product  SaturateOnIntegerOverflow=on  InputSameDT=on  OutDataTypeStr=Inherit: Same as first input
  Product5 : Product  SaturateOnIntegerOverflow=on  InputSameDT=on  OutDataTypeStr=Inherit: Same as first input
  RPM to rad/s : Gain  Commented=on  Gain=pi/30
  Sign : Signum
  Sum : Sum  SaturateOnIntegerOverflow=on  InputSameDT=on  OutDataTypeStr=Inherit: Same as first input
  Sum1 : Sum  Inputs=-+  SaturateOnIntegerOverflow=on  InputSameDT=on  OutDataTypeStr=Inherit: Same as first input
  Switch : Switch  SaturateOnIntegerOverflow=on
  Switch1 : Switch  SaturateOnIntegerOverflow=on
  cst : Constant
  max torque : Outport
  wires:
  Heat index/1(Heat index) -> Product2/2, Sum1/1
  cst/1 -> Sum1/2
  Product3/1 -> Sum/2
  Sum1/1 -> Product3/1
  Product2/1 -> Sum/1
  Switch1/1 -> Product3/2
  Switch/1 -> Heat index/1(cont torque), Product2/1
  Peak trq max - Regen/1 -> Switch1/3
  Cont trq max - Regen/1 -> Switch/3
  Cont trq max - Motoring/1 -> Switch/1
  torque/1 -> Heat index/2(torque)
  Abs/1 -> Product5/2
  Sum/1 -> Abs/1, Sign/1
  Product5/1 -> max torque/1
  Sign/1 -> Product5/1
  Memory/1 -> Cont trq max - Motoring/1, Cont trq max - Regen/1, Peak trq max - Motoring1/1, Peak trq max - Regen/1
  speed/1 -> Memory/1
  Constant/1 -> Divide/1
  RPM to rad/s/1 -> Divide by zero/1(In1)
  Abs2/1 -> 2-D Lookup Table/2
  Abs1/1 -> 2-D Lookup Table/1
  2-D Lookup Table/1 -> Gain2/1
  Gain2/1 -> Divide/2
  Req/1 -> Switch/2, Switch1/2
  Divide by zero/1(Out1) -> Divide/3
  Peak trq max - Motoring1/1 -> Switch1/1

== system Clutchless_P2_Parallel/Camaro Plant Model/E-Machine/Soft MCU/Torque Calculation2/max torque  ==
  Req : Inport
  speed : Inport  Port=2
  torque : Inport  Port=3
  2-D Lookup Table : Lookup_n-D  Commented=on  BreakpointsForDimension1=mot.plant.init.eff_trq.idx2_trq  BreakpointsForDimension2=mot.plant.init.eff_trq.idx1_spd  Table=mot.plant.init.eff_trq.map  InternalRulePriority=Speed  RndMeth=Simplest  InputSameDT=on
  Abs : Abs  SaturateOnIntegerOverflow=on
  Abs1 : Abs  Commented=on
  Abs2 : Abs  Commented=on
  Constant : Constant  Commented=on  Value=84500
  Cont trq max - Motoring : Lookup  InputValues=mot.plant.init.motor.trq_cont.idx1_spd  Table=mot.plant.init.motor.trq_cont.map  LookUpMeth=Interpolation-Use End Values  SaturateOnIntegerOverflow=on
  Cont trq max - Regen : Lookup  InputValues=mot.plant.init.regen.trq_cont.idx1_spd  Table=mot.plant.init.regen.trq_cont.map  LookUpMeth=Interpolation-Use End Values  SaturateOnIntegerOverflow=on
  Divide : Product  Commented=on  Inputs=**/
  Divide by zero : Subsystem  Commented=on
  Gain2 : Gain  Commented=on  Gain=1/100
  Heat index : Subsystem
  Memory : Memory
  Peak trq max - Motoring : Lookup  Commented=on  InputValues=mot.plant.init.regen.trq_max.idx1_spd  Table=mot.plant.init.motor.trq_max.map  LookUpMeth=Interpolation-Use End Values  SaturateOnIntegerOverflow=on
  Peak trq max - Motoring1 : Lookup  InputValues=mot.plant.init.regen.trq_max.idx1_spd  Table=mot.plant.init.motor.trq_max.map  LookUpMeth=Interpolation-Use End Values  SaturateOnIntegerOverflow=on
  Peak trq max - Regen : Lookup  InputValues=mot.plant.init.regen.trq_max.idx1_spd  Table=mot.plant.init.regen.trq_max.map  LookUpMeth=Interpolation-Use End Values  SaturateOnIntegerOverflow=on
  Product2 : Product  SaturateOnIntegerOverflow=on  InputSameDT=on  OutDataTypeStr=Inherit: Same as first input
  Product3 : Product  SaturateOnIntegerOverflow=on  InputSameDT=on  OutDataTypeStr=Inherit: Same as first input
  Product5 : Product  SaturateOnIntegerOverflow=on  InputSameDT=on  OutDataTypeStr=Inherit: Same as first input
  RPM to rad/s : Gain  Commented=on  Gain=pi/30
  Sign : Signum
  Sum : Sum  SaturateOnIntegerOverflow=on  InputSameDT=on  OutDataTypeStr=Inherit: Same as first input
  Sum1 : Sum  Inputs=-+  SaturateOnIntegerOverflow=on  InputSameDT=on  OutDataTypeStr=Inherit: Same as first input
  Switch : Switch  SaturateOnIntegerOverflow=on
  Switch1 : Switch  SaturateOnIntegerOverflow=on
  cst : Constant
  max torque : Outport
  wires:
  Heat index/1(Heat index) -> Product2/2, Sum1/1
  cst/1 -> Sum1/2
  Product3/1 -> Sum/2
  Sum1/1 -> Product3/1
  Product2/1 -> Sum/1
  Switch1/1 -> Product3/2
  Switch/1 -> Heat index/1(cont torque), Product2/1
  Peak trq max - Regen/1 -> Switch1/3
  Cont trq max - Regen/1 -> Switch/3
  Cont trq max - Motoring/1 -> Switch/1
  torque/1 -> Heat index/2(torque)
  Abs/1 -> Product5/2
  Sum/1 -> Abs/1, Sign/1
  Product5/1 -> max torque/1
  Sign/1 -> Product5/1
  Memory/1 -> Cont trq max - Motoring/1, Cont trq max - Regen/1, Peak trq max - Motoring1/1, Peak trq max - Regen/1
  speed/1 -> Memory/1
  Constant/1 -> Divide/1
  RPM to rad/s/1 -> Divide by zero/1(In1)
  Abs2/1 -> 2-D Lookup Table/2
  Abs1/1 -> 2-D Lookup Table/1
  2-D Lookup Table/1 -> Gain2/1
  Gain2/1 -> Divide/2
  Req/1 -> Switch/2, Switch1/2
  Divide by zero/1(Out1) -> Divide/3
  Peak trq max - Motoring1/1 -> Switch1/1

== system Clutchless_P2_Parallel/Camaro Plant Model/E-Machine/Soft MCU/Torque Calculation3/Subsystem ==
  In1 : Inport
  In2 : Inport  Port=2
  In3 : Inport  Port=3
  Switch : Switch  Criteria=u2 > Threshold  ZeroCross=off
  Torq : Outport
  wires:
  In2/1 -> Switch/2
  In3/1 -> Switch/3
  In1/1 -> Switch/1
  Switch/1 -> Torq/1

== system Clutchless_P2_Parallel/Camaro Plant Model/E-Machine/Soft MCU/Torque Calculation3/Subsystem1 ==
  In1 : Inport
  In2 : Inport  Port=2
  In3 : Inport  Port=3
  Switch : Switch  Criteria=u2 > Threshold  ZeroCross=off
  Current : Outport
  wires:
  Switch/1 -> Current/1
  In1/1 -> Switch/1
  In3/1 -> Switch/3
  In2/1 -> Switch/2

== system Clutchless_P2_Parallel/Camaro Plant Model/E-Machine/Soft MCU/Torque Calculation3/max torque  ==
  Req : Inport
  speed : Inport  Port=2
  torque : Inport  Port=3
  2-D Lookup Table : Lookup_n-D  Commented=on  BreakpointsForDimension1=mot.plant.init.eff_trq.idx2_trq  BreakpointsForDimension2=mot.plant.init.eff_trq.idx1_spd  Table=mot.plant.init.eff_trq.map  InternalRulePriority=Speed  RndMeth=Simplest  InputSameDT=on
  Abs : Abs  ZeroCross=off  SaturateOnIntegerOverflow=on
  Abs1 : Abs  Commented=on
  Abs2 : Abs  Commented=on
  Constant : Constant  Commented=on  Value=84500
  Cont trq max - Motoring : Lookup  InputValues=mot.plant.init.motor.trq_cont.idx1_spd  Table=mot.plant.init.motor.trq_cont.map  LookUpMeth=Interpolation-Use End Values  SaturateOnIntegerOverflow=on
  Cont trq max - Regen : Lookup  InputValues=mot.plant.init.regen.trq_cont.idx1_spd  Table=mot.plant.init.regen.trq_cont.map  LookUpMeth=Interpolation-Use End Values  SaturateOnIntegerOverflow=on
  Divide : Product  Commented=on  Inputs=**/
  Divide by zero : Subsystem  Commented=on
  Gain2 : Gain  Commented=on  Gain=1/100
  Heat index : Subsystem
  Peak trq max - Motoring : Lookup  Commented=on  InputValues=mot.plant.init.regen.trq_max.idx1_spd  Table=mot.plant.init.motor.trq_max.map  LookUpMeth=Interpolation-Use End Values  SaturateOnIntegerOverflow=on
  Peak trq max - Motoring1 : Lookup  InputValues=mot.plant.init.regen.trq_max.idx1_spd  Table=mot.plant.init.motor.trq_max.map  LookUpMeth=Interpolation-Use End Values  SaturateOnIntegerOverflow=on
  Peak trq max - Regen : Lookup  InputValues=mot.plant.init.regen.trq_max.idx1_spd  Table=mot.plant.init.regen.trq_max.map  LookUpMeth=Interpolation-Use End Values  SaturateOnIntegerOverflow=on
  Product2 : Product  SaturateOnIntegerOverflow=on  InputSameDT=on  OutDataTypeStr=Inherit: Same as first input
  Product3 : Product  SaturateOnIntegerOverflow=on  InputSameDT=on  OutDataTypeStr=Inherit: Same as first input
  Product5 : Product  SaturateOnIntegerOverflow=on  InputSameDT=on  OutDataTypeStr=Inherit: Same as first input
  RPM to rad/s : Gain  Commented=on  Gain=pi/30
  Scope : Scope
  Sign : Signum  ZeroCross=off
  Sum : Sum  SaturateOnIntegerOverflow=on  InputSameDT=on  OutDataTypeStr=Inherit: Same as first input
  Sum1 : Sum  Inputs=-+  SaturateOnIntegerOverflow=on  InputSameDT=on  OutDataTypeStr=Inherit: Same as first input
  Switch : Switch  SaturateOnIntegerOverflow=on
  Switch1 : Switch  SaturateOnIntegerOverflow=on
  cst : Constant
  max torque : Outport
  wires:
  Heat index/1(Heat index) -> Product2/2, Sum1/1
  cst/1 -> Sum1/2
  Product3/1 -> Sum/2
  Sum1/1 -> Product3/1
  Product2/1 -> Sum/1
  Switch1/1 -> Product3/2
  Switch/1 -> Heat index/1(cont torque), Product2/1
  Peak trq max - Regen/1 -> Switch1/3
  Cont trq max - Regen/1 -> Switch/3
  Cont trq max - Motoring/1 -> Switch/1
  torque/1 -> Heat index/2(torque)
  Abs/1 -> Product5/2
  Sum/1 -> Abs/1, Sign/1
  Product5/1 -> Scope/1, max torque/1
  Sign/1 -> Product5/1
  speed/1 -> Cont trq max - Motoring/1, Cont trq max - Regen/1, Peak trq max - Motoring1/1, Peak trq max - Regen/1
  Constant/1 -> Divide/1
  RPM to rad/s/1 -> Divide by zero/1(In1)
  Abs2/1 -> 2-D Lookup Table/2
  Abs1/1 -> 2-D Lookup Table/1
  2-D Lookup Table/1 -> Gain2/1
  Gain2/1 -> Divide/2
  Req/1 -> Switch/2, Switch1/2
  Divide by zero/1(Out1) -> Divide/3
  Peak trq max - Motoring1/1 -> Switch1/1

== system Clutchless_P2_Parallel/Clutchless_HSC/HSC/Camaro Fault Detection/Component Diagnostic/Driver Input Diagnostic ==
  note: Driver_CompStatus
      | 1 = Component Online
      | 0 = Component Offline
  note: APP1
      | APP2
      | BPP
      | Driver Component Status
      |
      | 1
      | 1
      | 1
      | 1
      |
      | 0
      | 1
      | 1
      | 1
      |
      | 1
      | 0
      | 1
      | 1
      |
      | 0
      | 0
      | 1
      | 0
      |
      | 1
      | 1
      | 0
      | 0
      |
      | 0
      | 0
      | 0
      | 0
  In1 : Inport
  Bus Selector : BusSelector  OutputSignals=Driver_SigDiag.Drv_APP1_[%]_SigValid,Driver_SigDiag.Drv_APP2_[%]_SigValid,Driver_SigDiag.Drv_APP_Agree,Driver_SigDiag.Drv_BPP_[%]_SigValid,Driver_SigDiag.Drv_KeyPos_[0 3]_SigValid,Driver_SigDiag.Drv_PRNDL_SigValid,Driver_SigDiag.Brake_Failed
  Driver_Input_Diag : Stateflow chart  TreatAsAtomicUnit=on
  Logical Operator : Logic  Inputs=3  AllPortsSameDT=off  OutDataTypeStr=boolean
  Out1 : Outport
  wires:
  In1/1 -> Bus Selector/1
  Bus Selector/1 -> Logical Operator/1  "<Drv_APP1_[%]_SigValid>"
  Bus Selector/2 -> Logical Operator/2  "<Drv_APP2_[%]_SigValid>"
  Bus Selector/4 -> Driver_Input_Diag/2(Drv_BPP_SigValid)  "<Drv_BPP_[%]_SigValid>"
  Driver_Input_Diag/1(Driver_Input_Status) -> Out1/1  "Driver_Input_Status"
  Logical Operator/1 -> Driver_Input_Diag/1(APP_Valid)  "APP_Valid"
  Bus Selector/3 -> Logical Operator/3  "<Drv_APP_Agree>"
  Bus Selector/5 -> Driver_Input_Diag/3(KeyPos)  "<Drv_KeyPos_[0 3]_SigValid>"
  Bus Selector/6 -> Driver_Input_Diag/4(PRNDL)  "<Drv_PRNDL_SigValid>"
  Bus Selector/7 -> Driver_Input_Diag/5(BrakeFail)  "<Brake_Failed>"

== system Clutchless_P2_Parallel/Clutchless_HSC/HSC/Camaro Fault Detection/Component Diagnostic/ESS Component Diagnostic ==
  note: (Need modify)
  In1 : Inport
  BMS_CompDiag1 : Stateflow chart  TreatAsAtomicUnit=on
  Bus Selector : BusSelector  OutputSignals=ESS_SigDiag.BMS_RollingAliveActive_SigValid,ESS_SigDiag.BMS_contactorsFailed_Detected,ESS_SigDiag.BMS_essTemp_[degC]_SigValid,ESS_SigDiag.essTempRange[0_4],ESS_SigDiag.BMS_essSOC_0_1_SigValid,ESS_SigDiag.essTempRange[0_4],ESS_SigDiag.essCur_A_SigValid,ESS_SigDiag.BMSgdf_SigValid,Driver_SigDiag.Drv_KeyPos_[0 3]_SigValid
  Compare To Zero : simulink/Logic and Bit Operations/Compare To Zero  relop===  OutDataTypeStr=boolean
  Data Type Conversion : DataTypeConversion
  HVessFltReset : Constant
  Logical Operator : Logic  Operator=OR  AllPortsSameDT=off  OutDataTypeStr=boolean
  Logical Operator1 : Logic  AllPortsSameDT=off  OutDataTypeStr=boolean
  Terminator : Terminator
  Terminator1 : Terminator
  Out1 : Outport
  wires:
  In1/1 -> Bus Selector/1
  Bus Selector/1 -> BMS_CompDiag1/1(BMS_RollingAliveActive_SigValid)  "<BMS_RollingAliveActive_SigValid>"
  Bus Selector/2 -> [contactorsFailed_Detected], BMS_CompDiag1/2(BMS_contactorsFailed_SigValid)  "<BMS_contactorsFailed_Detected>"
  BMS_CompDiag1/1(BMS_Status) -> Out1/1  "BMS_Status"
  Bus Selector/4 -> Terminator/1  "<essTempRange[0_4]>"
  Bus Selector/3 -> Data Type Conversion/1  "<BMS_essTemp_[degC]_SigValid>"
  Data Type Conversion/1 -> BMS_CompDiag1/3(BMS_essTemp_SigValid)  "BMS_essTemp_SigValid"
  Bus Selector/5 -> BMS_CompDiag1/4(BMS_essSOC_0_1_SigValid)  "<BMS_essSOC_0_1_SigValid>"
  Bus Selector/6 -> Terminator1/1  "<essTempRange[0_4]>"
  Bus Selector/7 -> BMS_CompDiag1/5(essCur_A_SigValid)  "<essCur_A_SigValid>"
  Bus Selector/9 -> Compare To Zero/1  "<Drv_KeyPos_[0 3]_SigValid>"
  Compare To Zero/1 -> Logical Operator/1
  HVessFltReset/1 -> Logical Operator/2
  Logical Operator/1 -> BMS_CompDiag1/7(ClearFault)
  Bus Selector/8 -> Logical Operator1/2  "<BMSgdf_SigValid>"
  Logical Operator1/1 -> BMS_CompDiag1/6(ess_GroundFault)
  [contactorsFailed_Detected] -> Logical Operator1/1

== system Clutchless_P2_Parallel/Clutchless_HSC/HSC/Camaro Fault Detection/Component Diagnostic/Engine Component Diagnostic ==
  note: Eng_Torq_MsmchLevel
      | 1:Normal torque
      | 2: Limit max power
      | 3: Deliver creep torque
      | 4: offline
  note: ENGTRQ_MSMCH_Degraded_CP (40Nm): ENGTRQ_Degraded fault code.
      | ENGTRQ_MSMCH_LimpHome_CP (70Nm): ENGTRQ_LimpHome
      | ENGTRQ_MSMCH_ErrCritical_CP (100Nm): ENGTRQ_ErrCritical
  note: Eng_tempRange
      | 1: normal
      | 2: high range
      | 3:above max
  note: add the temperature, mismatch torquesignal and have different status to the component
  note: 0: component needs to be offline
      | 1: component needs torque plant to deliver creep torque
      | 2: component needs torque plant to limit maximum torque delivery
      | 3: component needs torque plant to operate normally
  note: Notes
  In1 : Inport
  Bus Selector : BusSelector  OutputSignals=Engine_SigDiag.ECMRollingAliveActive,Engine_SigDiag.engTrqCmdRecvd_SigValid,Engine_SigDiag.ECMTrqCmd_Nm,Engine_SigDiag.EngActStdyStTorq_Nm,Engine_SigDiag.EngRunAtValid,Engine_SigDiag.Engine_Speed_rpm_SigValid,Engine_SigDiag.Eng_TempValid,Engine_SigDiag.Eng_TempRange[123],Driver_SigDiag.Drv_KeyPos_[0 3]_SigValid
  Bus Selector1 : BusSelector  OutputSignals=Eng_Torque_Mismch_Critical
  Compare To Zero : simulink/Logic and Bit Operations/Compare To Zero  relop===  OutDataTypeStr=boolean
  ECM_CompDiag : Stateflow chart  TreatAsAtomicUnit=on
  Eng_FltReset : Constant
  Eng_Torq_MsmchLevel : Stateflow chart  Commented=on  TreatAsAtomicUnit=on
  Logical Operator : Logic  Operator=OR  AllPortsSameDT=off  OutDataTypeStr=boolean
  Override  engTrqCmd : Subsystem
  Terminator1 : Terminator
  TorqMismatch Detection : Subsystem
  Out1 : Outport
  Out2 : Outport  Port=2
  wires:
  In1/1 -> Bus Selector/1
  Bus Selector/1 -> ECM_CompDiag/1(ECM_RollingAliveActive)  "<ECMRollingAliveActive>"
  Bus Selector/2 -> Override  engTrqCmd/1(In1)  "<engTrqCmdRecvd_SigValid>"
  Bus Selector/6 -> ECM_CompDiag/4(Engine_Speed_rpm_SigValid)  "<Engine_Speed_rpm_SigValid>"
  ECM_CompDiag/1(ECM_Status) -> Out1/1  "ECM_Status"
  Compare To Zero/1 -> Logical Operator/1
  Eng_FltReset/1 -> Logical Operator/2
  Logical Operator/1 -> ECM_CompDiag/6(ClearFault)
  Bus Selector/9 -> Compare To Zero/1  "<Drv_KeyPos_[0 3]_SigValid>"
  Bus Selector/7 -> Terminator1/1  "<Eng_TempValid>"
  Bus Selector/8 -> ECM_CompDiag/5(Eng_TempRange_123)  "<Eng_TempRange[123]>"
  Bus Selector/3 -> TorqMismatch Detection/1(In1)  "<ECMTrqCmd_Nm>"
  Bus Selector/4 -> TorqMismatch Detection/2(In2)  "<EngActStdyStTorq_Nm>"
  Bus Selector/5 -> TorqMismatch Detection/3(In3)  "<EngRunAtValid>"
  TorqMismatch Detection/1(Eng_Torque_Mismch) -> Bus Selector1/1, Out2/1  "EngTrqMismchType"
  Bus Selector1/1 -> ECM_CompDiag/3(Eng_Torq_Msmch)  "<Eng_Torque_Mismch_Critical>"
  Override  engTrqCmd/1(Out1) -> ECM_CompDiag/2(engTrqCmdRecvd_SigValid)
